simulink model "Vehical_Safety_control"  (R2024a)
settings: Solver=FixedStepAuto  StartTime=0.0  StopTime=100  RelTol=1e-3
settings Model: Creator=balap  LastModifiedBy=balap

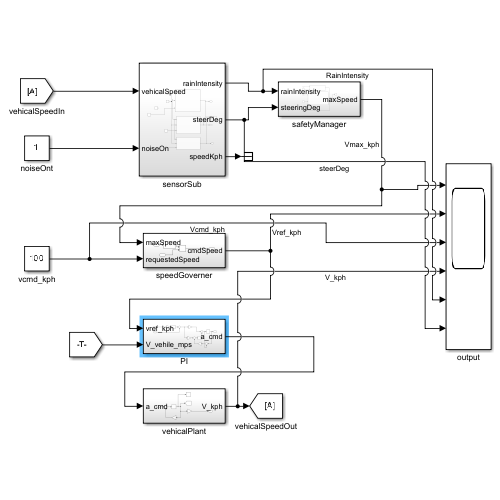
[thumbnail: Simulink's stored preview of the top-level diagram]
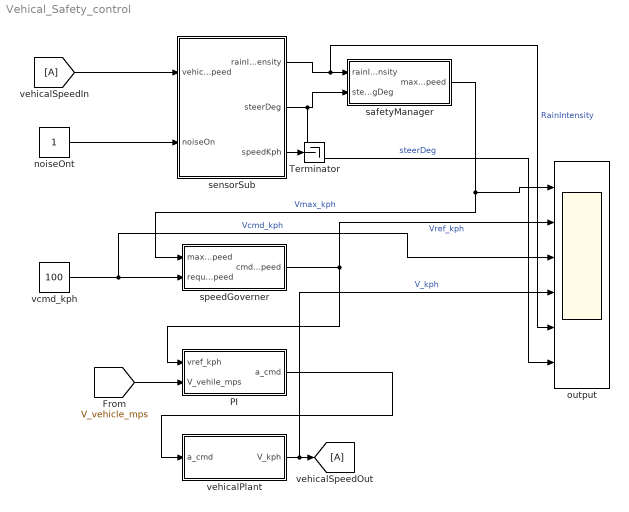
== system Vehical_Safety_control ==
  PI : Subsystem
  Terminator : Terminator
  noiseOnt : Constant
  output : Scope  NumInputPorts=6
  safetyManager : Subsystem
  sensorSub : Subsystem
  speedGoverner : Subsystem
  vcmd_kph : Constant  Value=100
  vehicalPlant : Subsystem
  vehicalSpeedIn : From
  vehicalSpeedOut : Goto
  wires:
  vehicalSpeedIn/1 -> sensorSub/1(vehicalSpeed)
  noiseOnt/1 -> sensorSub/2(noiseOn)
  sensorSub/1(rainIntensity) -> output/5, safetyManager/1(rainIntensity)  "RainIntensity"
  sensorSub/2(steerDeg) -> output/6, safetyManager/2(steeringDeg)  "steerDeg"
  safetyManager/1(maxSpeed) -> speedGoverner/1(maxSpeed), output/1  "Vmax_kph"
  sensorSub/3(speedKph) -> Terminator/1
  vcmd_kph/1 -> output/3, speedGoverner/2(requestedSpeed)  "Vcmd_kph"
  speedGoverner/1(cmdSpeed) -> PI/1(vref_kph), output/2  "Vref_kph"
  [V_vehicle_mps] -> PI/2(V_vehile_mps)
  PI/1(a_cmd) -> vehicalPlant/1(a_cmd)
  vehicalPlant/1(V_kph) -> output/4, vehicalSpeedOut/1  "V_kph"

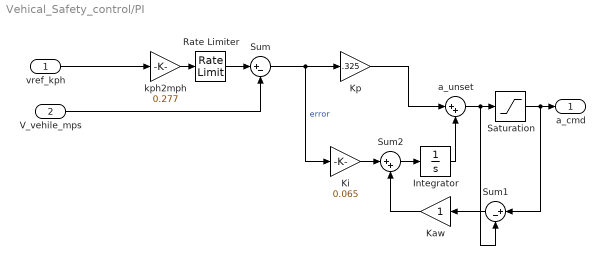
== system Vehical_Safety_control/PI ==
  vref_kph : Inport
  V_vehile_mps : Inport  Port=2
  Integrator : Integrator
  Kaw : Gain
  Ki : Gain  Gain=0.065
  Kp : Gain  Gain=.325
  Rate Limiter : RateLimiter  RisingSlewLimit=2  FallingSlewLimit=-4  SampleTimeMode=inherited
  Saturation : Saturate  UpperLimit=2.5  LowerLimit=-4
  Sum : Sum  Inputs=|+-
  Sum1 : Sum  Inputs=|+-
  Sum2 : Sum  Inputs=|++
  a_unset : Sum  Inputs=|++
  kph2mph : Gain  Gain=0.277
  a_cmd : Outport
  wires:
  vref_kph/1 -> kph2mph/1
  V_vehile_mps/1 -> Sum/2
  Sum/1 -> Ki/1, Kp/1  "error"
  Kp/1 -> a_unset/1
  Integrator/1 -> a_unset/2
  a_unset/1 -> Sum1/2, Saturation/1
  Saturation/1 -> Sum1/1, a_cmd/1
  Sum1/1 -> Kaw/1
  Ki/1 -> Sum2/1
  Kaw/1 -> Sum2/2
  Sum2/1 -> Integrator/1
  kph2mph/1 -> Rate Limiter/1
  Rate Limiter/1 -> Sum/1

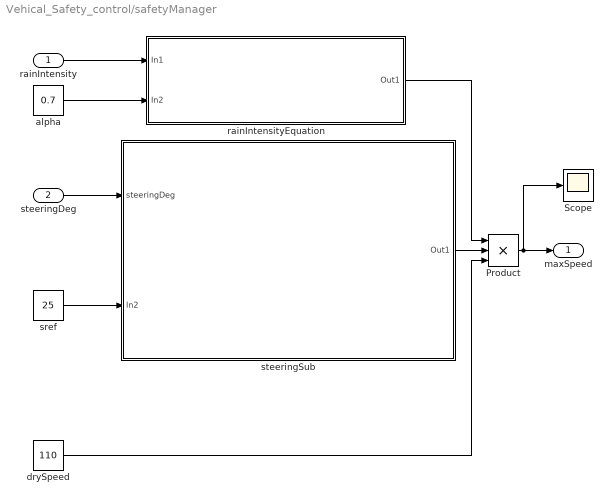
== system Vehical_Safety_control/safetyManager ==
  rainIntensity : Inport
  steeringDeg : Inport  Port=2
  Product : Product  Inputs=3
  Scope : Scope
  alpha : Constant  Value=0.7
  drySpeed : Constant  Value=110
  rainIntensityEquation : Subsystem
  sref : Constant  Value=25
  steeringSub : Subsystem
  maxSpeed : Outport
  wires:
  rainIntensity/1 -> rainIntensityEquation/1(In1)
  alpha/1 -> rainIntensityEquation/2(In2)
  sref/1 -> steeringSub/2(In2)
  Product/1 -> Scope/1, maxSpeed/1
  steeringSub/1(Out1) -> Product/2
  rainIntensityEquation/1(Out1) -> Product/1
  drySpeed/1 -> Product/3
  steeringDeg/1 -> steeringSub/1(steeringDeg)

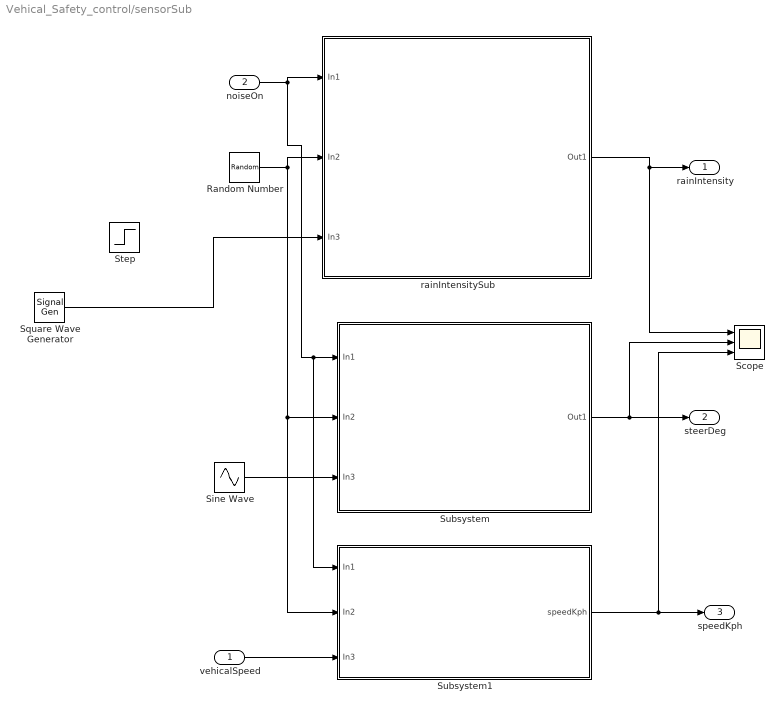
== system Vehical_Safety_control/sensorSub ==
  vehicalSpeed : Inport
  noiseOn : Inport  Port=2
  Random Number : RandomNumber  Variance=0.0005  Seed=123  SampleTime=0.01
  Scope : Scope  NumInputPorts=3
  Sine Wave : Sin  Amplitude=10  Frequency=0.02  SampleTime=0
  Square Wave Generator : SignalGenerator  WaveForm=square  Amplitude=0.7  Frequency=0.045  Units=rad/sec
  Step : Step  Time=12  After=0.7  SampleTime=0
  Subsystem : Subsystem
  Subsystem1 : Subsystem
  rainIntensitySub : Subsystem
  rainIntensity : Outport
  steerDeg : Outport  Port=2
  speedKph : Outport  Port=3
  wires:
  noiseOn/1 -> Subsystem1/1(In1), Subsystem/1(In1), rainIntensitySub/1(In1)
  Random Number/1 -> Subsystem1/2(In2), Subsystem/2(In2), rainIntensitySub/2(In2)
  rainIntensitySub/1(Out1) -> rainIntensity/1, Scope/1
  Subsystem/1(Out1) -> Scope/2, steerDeg/1
  vehicalSpeed/1 -> Subsystem1/3(In3)
  Subsystem1/1(speedKph) -> Scope/3, speedKph/1
  Sine Wave/1 -> Subsystem/3(In3)
  Square Wave Generator/1 -> rainIntensitySub/3(In3)

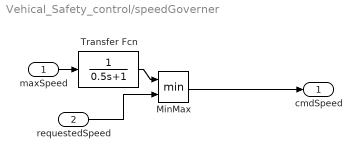
== system Vehical_Safety_control/speedGoverner ==
  maxSpeed : Inport
  requestedSpeed : Inport  Port=2
  MinMax : MinMax  Inputs=2
  Transfer Fcn : TransferFcn  Denominator=[0.5 1]
  cmdSpeed : Outport
  wires:
  requestedSpeed/1 -> MinMax/2
  MinMax/1 -> cmdSpeed/1
  maxSpeed/1 -> Transfer Fcn/1
  Transfer Fcn/1 -> MinMax/1

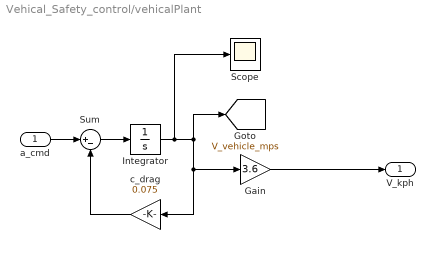
== system Vehical_Safety_control/vehicalPlant ==
  a_cmd : Inport
  Gain : Gain  Gain=3.6
  Integrator : Integrator
  Scope : Scope
  Sum : Sum  Inputs=|+-
  c_drag : Gain  Gain=0.075
  V_kph : Outport
  tag scope: V_vehicle_mps=global
  wires:
  a_cmd/1 -> Sum/1
  Sum/1 -> Integrator/1
  Integrator/1 -> Scope/1, Gain/1, c_drag/1, [V_vehicle_mps]
  c_drag/1 -> Sum/2
  Gain/1 -> V_kph/1

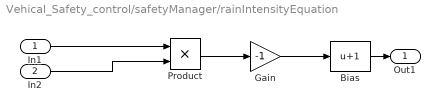
== system Vehical_Safety_control/safetyManager/rainIntensityEquation ==
  In1 : Inport
  In2 : Inport  Port=2
  Bias : Bias  Bias=1  SaturateOnIntegerOverflow=off
  Gain : Gain  Gain=-1
  Product : Product
  Out1 : Outport
  wires:
  Product/1 -> Gain/1
  Gain/1 -> Bias/1
  In1/1 -> Product/1
  In2/1 -> Product/2
  Bias/1 -> Out1/1

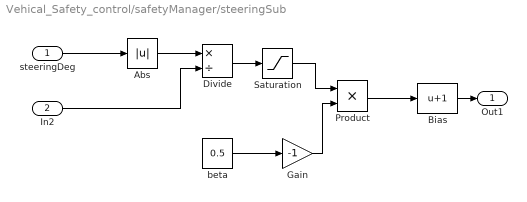
== system Vehical_Safety_control/safetyManager/steeringSub ==
  steeringDeg : Inport
  In2 : Inport  Port=2
  Abs : Abs  SaturateOnIntegerOverflow=off
  Bias : Bias  Bias=1  SaturateOnIntegerOverflow=off
  Divide : Product  Inputs=*/
  Gain : Gain  Gain=-1
  Product : Product
  Saturation : Saturate  UpperLimit=1  LowerLimit=0
  beta : Constant  Value=0.5
  Out1 : Outport
  wires:
  In2/1 -> Divide/2
  Bias/1 -> Out1/1
  Abs/1 -> Divide/1
  Divide/1 -> Saturation/1
  Saturation/1 -> Product/1
  Product/1 -> Bias/1
  beta/1 -> Gain/1
  steeringDeg/1 -> Abs/1
  Gain/1 -> Product/2

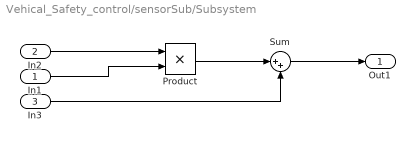
== system Vehical_Safety_control/sensorSub/Subsystem ==
  In1 : Inport
  In2 : Inport  Port=2
  In3 : Inport  Port=3
  Product : Product
  Sum : Sum  Inputs=|++
  Out1 : Outport
  wires:
  Product/1 -> Sum/1
  In1/1 -> Product/2
  Sum/1 -> Out1/1
  In2/1 -> Product/1
  In3/1 -> Sum/2

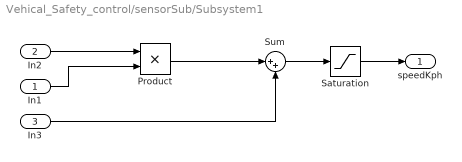
== system Vehical_Safety_control/sensorSub/Subsystem1 ==
  In1 : Inport
  In2 : Inport  Port=2
  In3 : Inport  Port=3
  Product : Product
  Saturation : Saturate  UpperLimit=inf  LowerLimit=0
  Sum : Sum  Inputs=|++
  speedKph : Outport
  wires:
  Product/1 -> Sum/1
  In1/1 -> Product/2
  Sum/1 -> Saturation/1
  In3/1 -> Sum/2
  Saturation/1 -> speedKph/1
  In2/1 -> Product/1

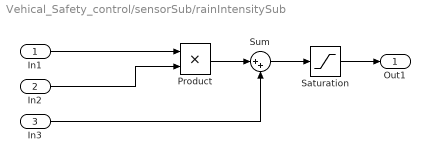
== system Vehical_Safety_control/sensorSub/rainIntensitySub ==
  In1 : Inport
  In2 : Inport  Port=2
  In3 : Inport  Port=3
  Product : Product
  Saturation : Saturate  UpperLimit=1  LowerLimit=0
  Sum : Sum  Inputs=|++
  Out1 : Outport
  wires:
  In3/1 -> Sum/2
  Product/1 -> Sum/1
  In2/1 -> Product/2
  Sum/1 -> Saturation/1
  In1/1 -> Product/1
  Saturation/1 -> Out1/1
